simulink model "PID_controller"  (R2020b)
settings: Solver=VariableStepAuto  StartTime=0.0  StopTime=10.0  RelTol=1e-3
settings Model: Creator=kshir  LastModifiedBy=kshir
settings DataIOCC: SaveOutput=off  SaveTime=off

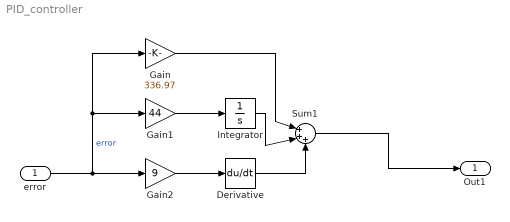
== system PID_controller ==
  error : Inport  OutDataTypeStr=double  PortDimensions=1  SampleTime=0
  Derivative : Derivative
  Gain : Gain  Gain=336.97
  Gain1 : Gain  Gain=44
  Gain2 : Gain  Gain=9
  Integrator : Integrator
  Sum1 : Sum  Inputs=|+++
  Out1 : Outport  OutDataTypeStr=double  PortDimensions=1  SampleTime=0
  wires:
  Integrator/1 -> Sum1/2
  Gain2/1 -> Derivative/1
  Derivative/1 -> Sum1/3
  error/1 -> Gain2/1, Gain1/1, Gain/1  "error"
  Sum1/1 -> Out1/1
  Gain/1 -> Sum1/1
  Gain1/1 -> Integrator/1
